simulink library "filteredPIDController_ul"  (R2018b)
settings: Solver=VariableStepAuto  StartTime=0.0  StopTime=10.0  RelTol=1e-3
undefined symbols (not defined in the file or in its folder): kd, ki, kp, tau
settings Model: Creator=mcobb  LastModifiedBy=mcobb

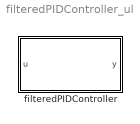
== system filteredPIDController_ul ==
  filteredPIDController : Subsystem  mask{kp=kp, ki=ki, kd=kd, Value=tau}
      mask prompts: kp "Proportional Gain, kp"; ki "Integral Gain, ki"; kd "Derivative Gain, kd"; Value "Time Constant, s"
      mask TypeOptions kp: kp/Gain
      mask TypeOptions ki: ki/Gain
      mask TypeOptions kd: kd/Gain
      mask TypeOptions Value: tau/Value

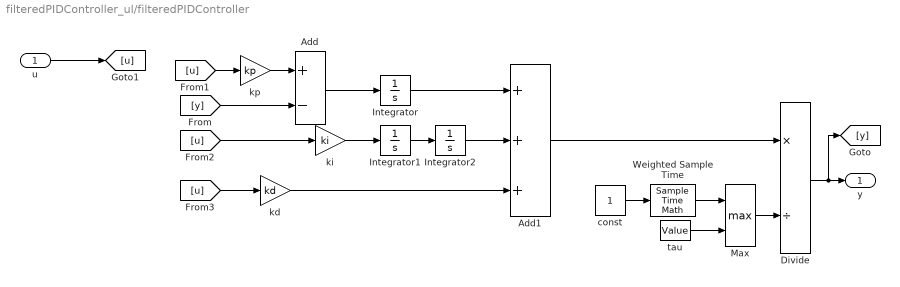
== system filteredPIDController_ul/filteredPIDController ==
  u : Inport  PortDimensions=1
  Add : Sum  Inputs=+-
  Add1 : Sum  Inputs=+++
  Divide : Product  Inputs=*/
  Integrator : Integrator
  Integrator1 : Integrator
  Integrator2 : Integrator
  Max : MinMax  Function=max  Inputs=2
  Weighted Sample Time : SampleTimeMath  TsampMathOp=Ts Only
  const : Constant
  kd : Gain  Gain=kd
  ki : Gain  Gain=ki
  kp : Gain  Gain=kp
  tau : Constant  Value=Value
  y : Outport  PortDimensions=1
  wires:
  u/1 -> [u]
  kp/1 -> Add/1
  [y] -> Add/2
  Add/1 -> Integrator/1
  [u] -> kp/1
  Max/1 -> Divide/2
  tau/1 -> Max/2
  Integrator1/1 -> Integrator2/1
  ki/1 -> Integrator1/1
  [u] -> ki/1
  [u] -> kd/1
  Integrator2/1 -> Add1/2
  Integrator/1 -> Add1/1
  kd/1 -> Add1/3
  Add1/1 -> Divide/1
  Divide/1 -> [y], y/1
  Weighted Sample Time/1 -> Max/1
  const/1 -> Weighted Sample Time/1
